simulink model "bungee_blocks"  (R2021b)
settings: Solver=ode45  StartTime=0.0  StopTime=100  MaxStep=0.01  RelTol=1e-3
values from neighbouring files (symbols this model uses):
  a1 = 1    [bungeescript.m]
  a2 = 1    [bungeescript.m]
  g = 10    [bungeescript.m]
  m = 90    [bungeescript.m]
undefined symbols (not defined in the file or in its folder): k
settings Model: Creator=SeoJiHun  LastModifiedBy=SeoJiHun

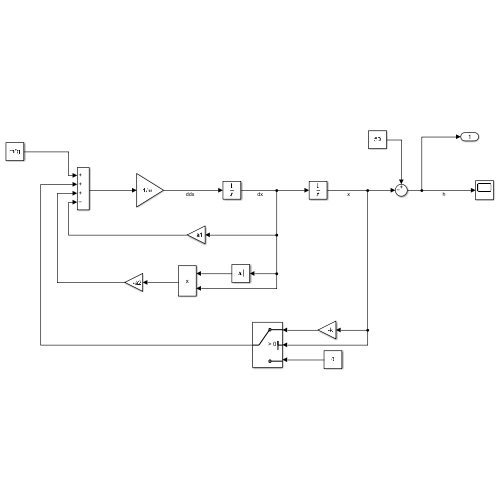
[thumbnail: Simulink's stored preview of the top-level diagram]
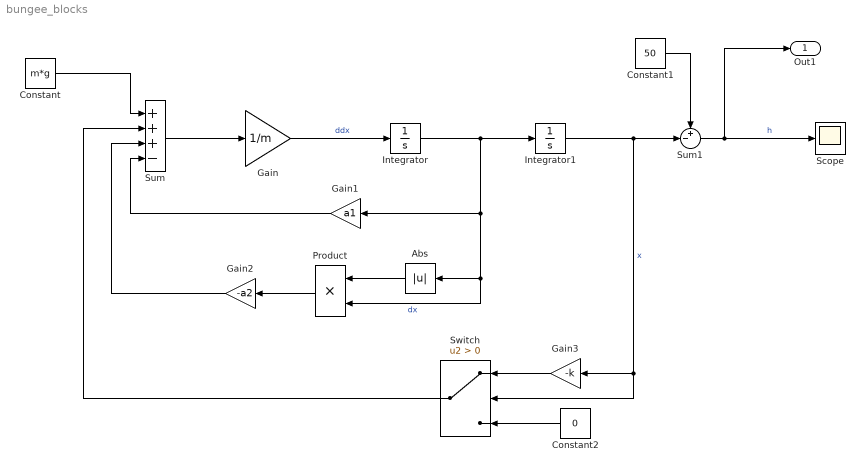
== system bungee_blocks ==
  Abs : Abs
  Constant : Constant  Value=m*g
  Constant1 : Constant  Value=50
  Constant2 : Constant  Value=0
  Gain : Gain  Gain=1/m
  Gain1 : Gain  Gain=a1
  Gain2 : Gain  Gain=-a2
  Gain3 : Gain  Gain=-k
  Integrator : Integrator
  Integrator1 : Integrator  InitialCondition=-30
  Product : Product
  Scope : Scope
  Sum : Sum  Inputs=+++-
  Sum1 : Sum  Inputs=+-|
  Switch : Switch  Criteria=u2 > Threshold
  Out1 : Outport
  wires:
  Gain/1 -> Integrator/1  "ddx"
  Integrator/1 -> Product/2, Abs/1, Gain1/1, Integrator1/1  "dx"
  Integrator1/1 -> Switch/2, Gain3/1, Sum1/2  "x"
  Constant1/1 -> Sum1/1
  Sum1/1 -> Out1/1, Scope/1  "h"
  Sum/1 -> Gain/1
  Gain1/1 -> Sum/4
  Abs/1 -> Product/1
  Product/1 -> Gain2/1
  Gain2/1 -> Sum/3
  Gain3/1 -> Switch/1
  Constant2/1 -> Switch/3
  Switch/1 -> Sum/2
  Constant/1 -> Sum/1
